simulink model "test_model"  (R2020b)
settings: Solver=FixedStepAuto  StartTime=0.0  StopTime=inf  RelTol=1e-3
libraries: DSX_Lib x5
settings Model: PacingRate=0.450000  Creator=16047  LastModifiedBy=16047

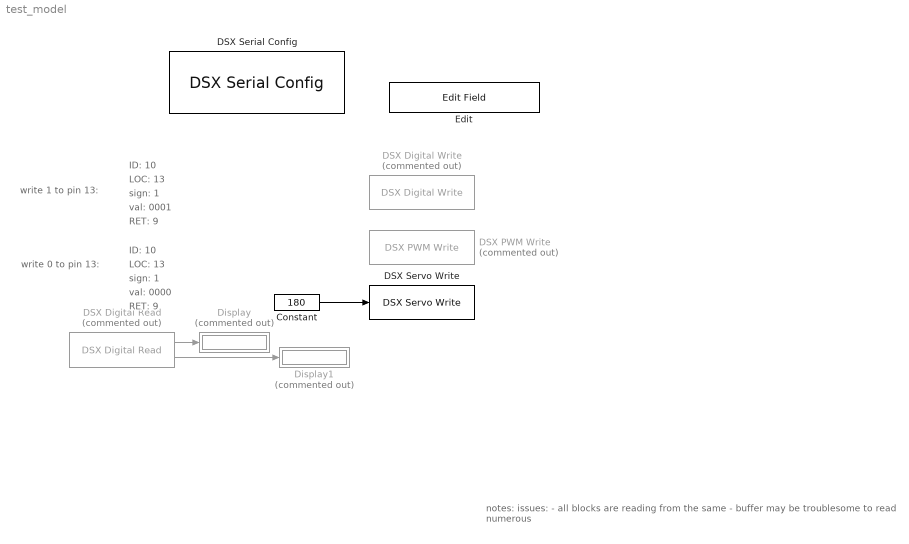
== system test_model ==
  note: notes:
      |
      | issues:
      | 	- all blocks are reading from the same
      | - buffer
      | may be troublesome to read numerous
  note: write 0 to pin 13:
  note: write 1 to pin 13:
  note: ID: 10
  note: LOC: 13
  note: sign: 1
  note: val: 0001
  note: RET: 9
  note: ID: 10
  note: LOC: 13
  note: sign: 1
  note: val: 0000
  note: RET: 9
  Constant : Constant  Value=180
  DSX Digital Read : DSX_Lib/DSX Blocks/DSX Digital Read  Commented=on  receive_func=GPIO  receive_loc=2
      settings: SourceProductName=DSX Library
  DSX Digital Write : DSX_Lib/DSX Blocks/DSX Digital Write  Commented=on  dtype=GPIO  gpio_pin=13  pwm_pin=8  pwm_freq=30
      settings: SourceProductName=DSX Library
  DSX PWM Write : DSX_Lib/DSX Blocks/DSX PWM Write  Commented=on  pwm_pin=3  pwm_freq=4000
      settings: SourceProductName=DSX Library
  DSX Serial Config : DSX_Lib/DSX Blocks/DSX Serial Config  ComPort=COM5  BaudRate=9600
      settings: SourceProductName=DSX Library
  DSX Servo Write : DSX_Lib/DSX Blocks/DSX Servo Write  servo_pin=16
      settings: SourceProductName=DSX Library
  Display : Display  Commented=on
  Display1 : Display  Commented=on
  Edit : EditField  LabelPosition=Hide  ShowInitialText=on  Alignment=Center
  wires:
  DSX Digital Read/1 -> Display/1
  DSX Digital Read/2 -> Display1/1
  Constant/1 -> DSX Servo Write/1
